simulink model "pid_tune"  (R2021a)
settings: Solver=ode4  StartTime=0.0  StopTime=T  FixedStep=step  RelTol=1e-3
values from neighbouring files (symbols this model uses):
  g = 9.81    [parameters.m]
  l = 0.1    [parameters.m]
  M = 2    [parameters.m]
  m = 1    [parameters.m]
settings Model: Creator=kpiek  LastModifiedBy=kpiek

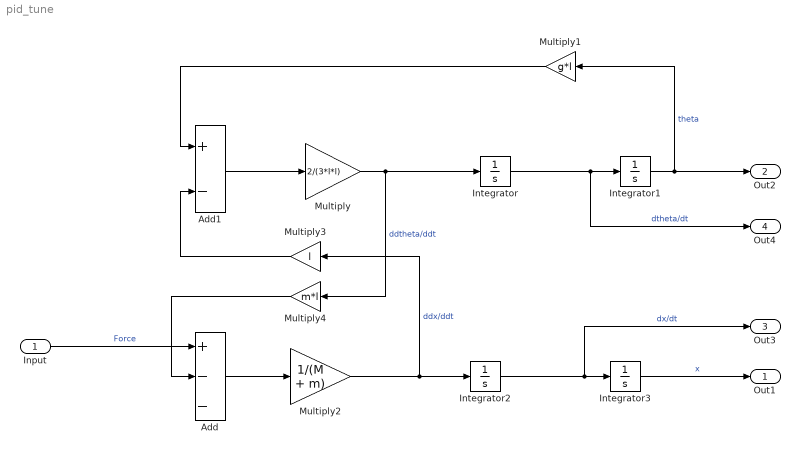
== system pid_tune ==
  Input : Inport
  Add : Sum  Inputs=+--
  Add1 : Sum  Inputs=+-
  Integrator{,1..3} (4 alike) : Integrator
  Multiply : Gain  Gain=2/(3*l*l)
  Multiply1 : Gain  Gain=g*l
  Multiply2 : Gain  Gain=1/(M + m)
  Multiply3 : Gain  Gain=l
  Multiply4 : Gain  Gain=m*l
  Out1 : Outport
  Out2 : Outport  Port=2
  Out3 : Outport  Port=3
  Out4 : Outport  Port=4
  wires:
  Add1/1 -> Multiply/1
  Multiply/1 -> Multiply4/1, Integrator/1  "ddtheta/ddt"
  Integrator/1 -> Out4/1, Integrator1/1  "dtheta/dt"
  Integrator1/1 -> Out2/1, Multiply1/1  "theta"
  Multiply1/1 -> Add1/1
  Input/1 -> Add/1  "Force"
  Add/1 -> Multiply2/1
  Multiply2/1 -> Multiply3/1, Integrator2/1  "ddx/ddt"
  Integrator2/1 -> Out3/1, Integrator3/1  "dx/dt"
  Integrator3/1 -> Out1/1  "x"
  Multiply3/1 -> Add1/2
  Multiply4/1 -> Add/2
